simulink model "P5_P"  (R2023b)
settings: Solver=VariableStepAuto  StartTime=0.0  StopTime=10.0  RelTol=1e-3
settings Model: Creator=Diego  LastModifiedBy=Diego

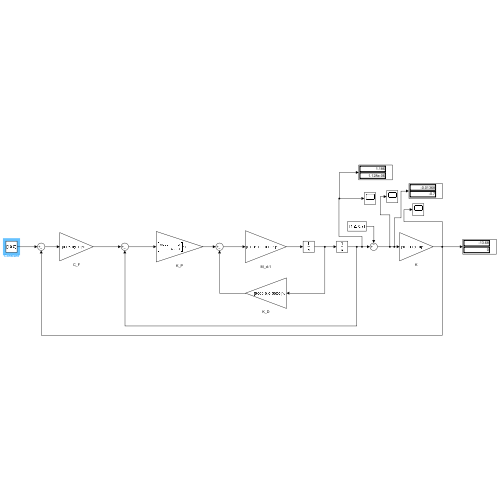
[thumbnail: Simulink's stored preview of the top-level diagram]
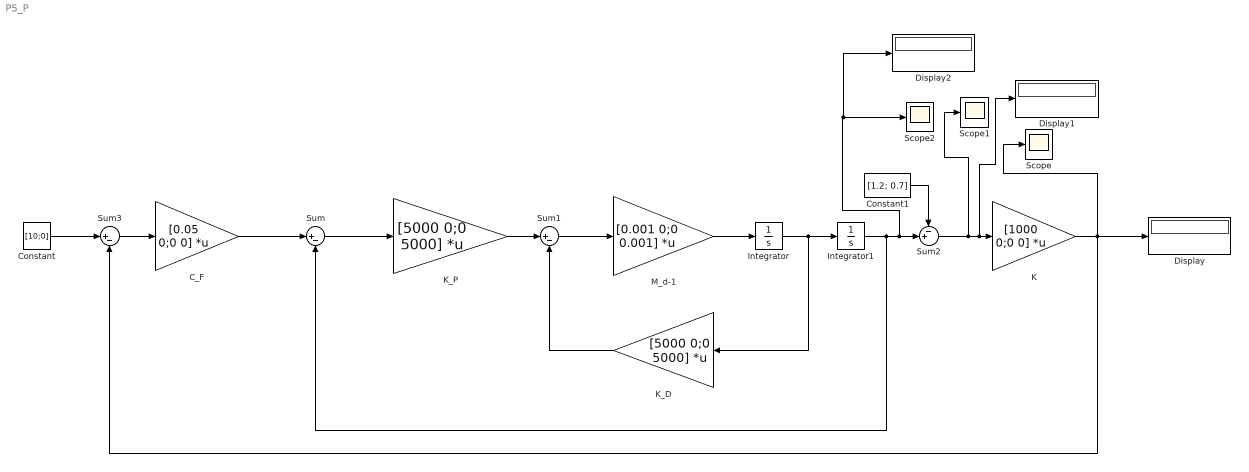
== system P5_P ==
  C_F : Gain  Gain=[0.05 0;0 0]  Multiplication=Matrix(K*u)
  Constant : Constant  Value=[10;0]
  Constant1 : Constant  Value=[1.2; 0.7]
  Display : Display
  Display1 : Display
  Display2 : Display
  Integrator : Integrator  InitialCondition=[0;0]
  Integrator1 : Integrator  InitialCondition=[1.3; 0.7]
  K : Gain  Gain=[1000 0;0 0]  Multiplication=Matrix(K*u)
  K_D : Gain  Gain=[5000 0;0 5000]  Multiplication=Matrix(K*u)
  K_P : Gain  Gain=[5000 0;0 5000]  Multiplication=Matrix(K*u)
  M_d-1 : Gain  Gain=[0.001 0;0 0.001]  Multiplication=Matrix(K*u)
  Scope : Scope
  Scope1 : Scope
  Scope2 : Scope
  Sum : Sum  Inputs=|+-
  Sum1 : Sum  Inputs=|+-
  Sum2 : Sum  Inputs=-+|
  Sum3 : Sum  Inputs=|+-
  wires:
  C_F/1 -> Sum/1
  Sum/1 -> K_P/1
  Sum1/1 -> M_d-1/1
  K_P/1 -> Sum1/1
  M_d-1/1 -> Integrator/1
  Integrator/1 -> K_D/1, Integrator1/1
  Integrator1/1 -> Display2/1, Scope2/1, Sum2/2, Sum/2
  Sum2/1 -> Scope1/1, Display1/1, K/1
  K/1 -> Scope/1, Sum3/2, Display/1
  Sum3/1 -> C_F/1
  Constant/1 -> Sum3/1
  Constant1/1 -> Sum2/1
  K_D/1 -> Sum1/2
